simulink subsystem "PieroAdry_HW"  (R2023b)
settings: Solver=VariableStepAuto  StartTime=0.0  StopTime=10.0  RelTol=1e-3
settings Model: Creator=johan  LastModifiedBy=adria

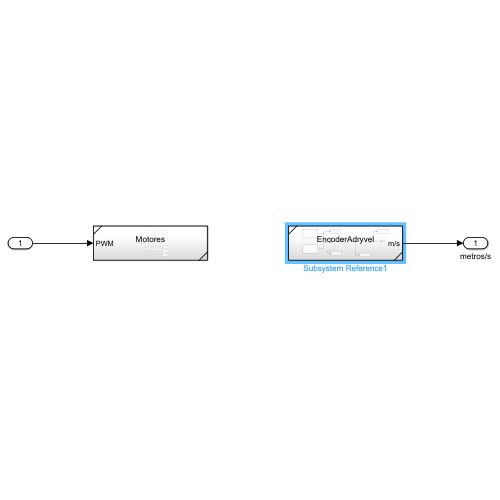
[thumbnail: Simulink's stored preview of the top-level diagram]
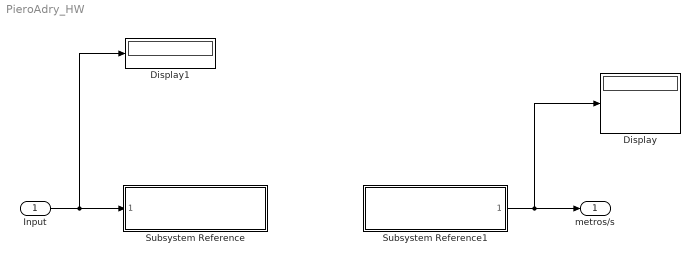
== system PieroAdry_HW ==
  Input : Inport  OutDataTypeStr=int16
  Display : Display
  Display1 : Display
  Subsystem Reference : Subsystem  ReferencedSubsystem=Motores
  Subsystem Reference1 : Subsystem  ReferencedSubsystem=EncoderAdryvel
  metros/s : Outport  OutDataTypeStr=double
  wires:
  Input/1 -> Subsystem Reference/1, Display1/1
  Subsystem Reference1/1 -> metros/s/1, Display/1
